simulink model "LQRSimulink"  (R2025b)
settings: Solver=VariableStepAuto  StartTime=0.0  StopTime=1000  RelTol=1e-3
undefined symbols (not defined in the file): A_long, B_ctrl, best_theta, K
libraries: aerolibwind2 x1
settings Model: Creator=leonardoleggeri  LastModifiedBy=leonardoleggeri

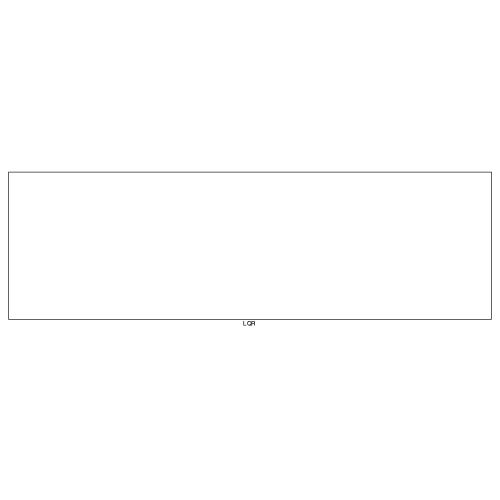
[thumbnail: Simulink's stored preview of the top-level diagram]
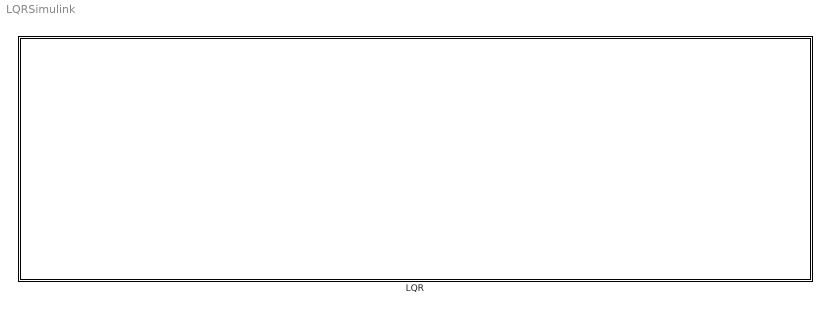
== system LQRSimulink ==
  LQR : Subsystem

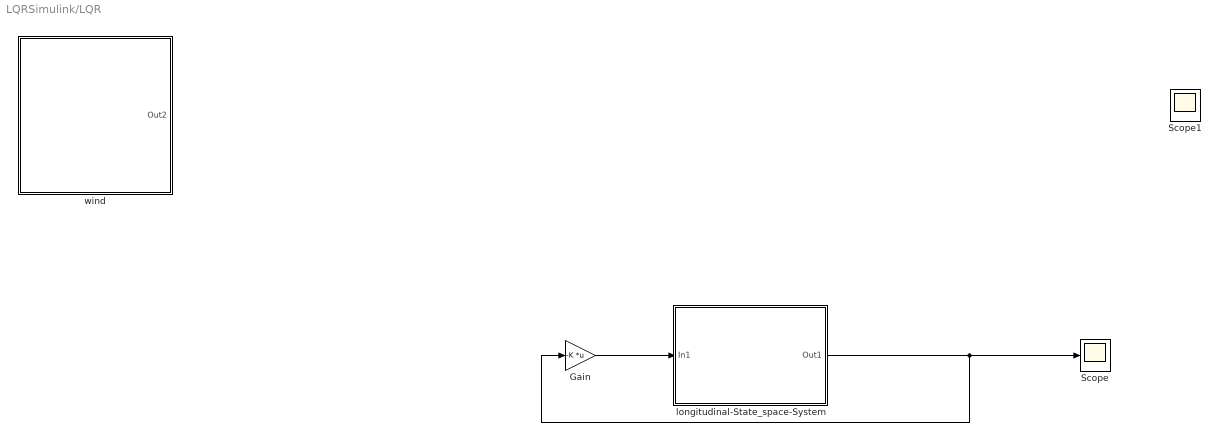
== system LQRSimulink/LQR ==
  Gain : Gain  Gain=-K  Multiplication=Matrix(K*u)
  Scope : Scope
      settings: ActiveDisplayYMinimum=-0.019323209618269076  ActiveDisplayYMaximum=0.019619008347149653
  Scope1 : Scope
      settings: ActiveDisplayYMinimum=-0.019323209618269076  ActiveDisplayYMaximum=0.019619008347149653  DataLoggingVariableName=ScopeData2
  longitudinal-State_space-System : Subsystem
      mask Display: image('F16_SCANG_InFlight.jpg');
  wind : Subsystem
  wires:
  longitudinal-State_space-System/1(Out1) -> Scope/1, Gain/1
  Gain/1 -> longitudinal-State_space-System/1(In1)

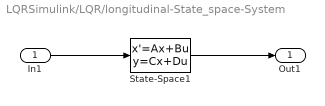
== system LQRSimulink/LQR/longitudinal-State_space-System ==
  In1 : Inport
  State-Space1 : StateSpace  A=A_long  B=B_ctrl  C=eye(4)  D=zeros(4,3)  InitialCondition=[5;0;0;0.08]
  Out1 : Outport
  wires:
  In1/1 -> State-Space1/1
  State-Space1/1 -> Out1/1

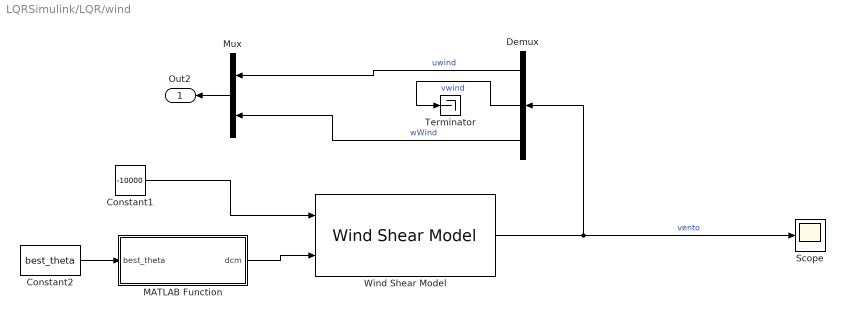
== system LQRSimulink/LQR/wind ==
  Constant1 : Constant  Value=-10000
  Constant2 : Constant  Value=best_theta
  Demux : Demux  Outputs=3
  MATLAB Function : MATLAB Function  TreatAsAtomicUnit=on
  Mux : Mux  Inputs=2
  Scope : Scope
      settings: ActiveDisplayYMinimum=-1.998657658680921  ActiveDisplayYMaximum=0.68071031120572645
  Terminator : Terminator
  Wind Shear Model : aerolibwind2/Wind Shear Model  units=Metric (MKS)  phase=Other  W_20=15  Wdeg=45
  Out2 : Outport
  wires:
  Mux/1 -> Out2/1
  Demux/1 -> Mux/1  "uwind"
  Constant1/1 -> Wind Shear Model/1
  Wind Shear Model/1 -> Scope/1, Demux/1  "vento"
  Demux/2 -> Terminator/1  "vwind"
  Demux/3 -> Mux/2  "wWind"
  Constant2/1 -> MATLAB Function/1(best_theta)
  MATLAB Function/1(dcm) -> Wind Shear Model/2

== matlab function LQRSimulink/LQR/wind/MATLAB Function ==
  data: best_theta input; dcm output
function dcm = calcola_dcm(best_theta)
    % La variabile in ingresso (best_theta) viene usata per calcolare la DCM
    dcm = [ cos(best_theta),  0, -sin(best_theta);
            0,                1,  0;
            sin(best_theta),  0,  cos(best_theta)];
end
